simulink model "AeroModel_v2point1"  (R2021a)
settings: Solver=ode4  StartTime=0.0  StopTime=10.0  FixedStep=0.0001  RelTol=1e-3
settings Model: Creator=jadg1  LastModifiedBy=jadg1

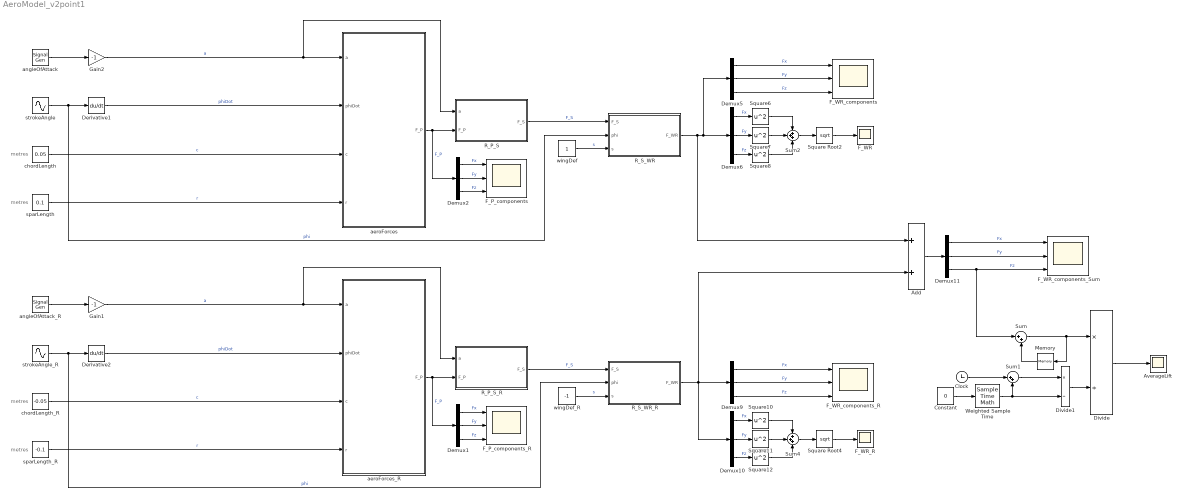
== system AeroModel_v2point1 ==
  note: metres
  note: metres
  note: metres
  note: metres
  Add : Sum
  AverageLift : Scope
  Clock : Clock
  Constant : Constant  Value=0
  Demux{1..2,5..6,9..11} (7 alike) : Demux  Outputs=3
  Derivative1 : Derivative
  Derivative2 : Derivative
  Divide : Product  Inputs=*/
  Divide1 : Product  Inputs=*/
  F_P_components : Scope  NumInputPorts=3
  F_P_components_R : Scope  NumInputPorts=3
  F_WR : Scope
  F_WR_R : Scope
  F_WR_components : Scope  NumInputPorts=3
  F_WR_components_R : Scope  NumInputPorts=3
  F_WR_components_Sum : Scope  NumInputPorts=3
  Gain1 : Gain  Gain=-1
  Gain2 : Gain  Gain=-1
  Memory : Memory
  R_P_S : MATLAB Function  TreatAsAtomicUnit=on
  R_P_S_R : MATLAB Function  TreatAsAtomicUnit=on
  R_S_WR : MATLAB Function  TreatAsAtomicUnit=on
  R_S_WR_R : MATLAB Function  TreatAsAtomicUnit=on
  Square Root2 : Sqrt  SaturateOnIntegerOverflow=on
  Square Root4 : Sqrt  SaturateOnIntegerOverflow=on
  Square{6..8,10..12} (6 alike) : Math  Operator=square  SaturateOnIntegerOverflow=on
  Sum : Sum  Inputs=|++
  Sum1 : Sum  Inputs=|++
  Sum2 : Sum  Inputs=+++
  Sum4 : Sum  Inputs=+++
  Weighted Sample Time : SampleTimeMath  TsampMathOp=Ts Only
  aeroForces : MATLAB Function  TreatAsAtomicUnit=on
  aeroForces_R : MATLAB Function  TreatAsAtomicUnit=on
  angleOfAttack : SignalGenerator  WaveForm=square  Amplitude=pi()/4  Frequency=30
  angleOfAttack_R : SignalGenerator  WaveForm=square  Amplitude=pi()/4  Frequency=30
  chordLength : Constant  Value=0.05
  chordLength_R : Constant  Value=-0.05
  sparLength : Constant  Value=0.1
  sparLength_R : Constant  Value=-0.1
  strokeAngle : Sin  Amplitude=pi()/2  Frequency=188.5  Phase=pi()/2  SampleTime=0
  strokeAngle_R : Sin  Amplitude=pi()/2  Frequency=188.5  Phase=pi()/2  SampleTime=0
  wingDef : Constant
  wingDef_R : Constant  Value=-1
  wires:
  Square11/1 -> Sum4/2
  sparLength/1 -> aeroForces/4(r)  "r"
  Demux1/3 -> F_P_components_R/3  "Fz"
  wingDef_R/1 -> R_S_WR_R/3(s)  "s"
  Derivative2/1 -> aeroForces_R/2(phiDot)  "phiDot"
  Demux10/1 -> Square10/1  "Fx"
  angleOfAttack_R/1 -> Gain1/1
  R_P_S/1(F_S) -> R_S_WR/1(F_S)  "F_S"
  Demux1/2 -> F_P_components_R/2  "Fy"
  Demux5/3 -> F_WR_components/3  "Fz"
  Demux2/3 -> F_P_components/3  "Fz"
  wingDef/1 -> R_S_WR/3(s)  "s"
  Demux10/2 -> Square11/1  "Fy"
  Gain2/1 -> R_P_S/1(a), aeroForces/1(a)  "a"
  R_S_WR_R/1(F_WR) -> Demux10/1, Demux9/1, Add/2
  Square10/1 -> Sum4/1
  Demux9/2 -> F_WR_components_R/2  "Fy"
  Sum4/1 -> Square Root4/1
  Demux10/3 -> Square12/1  "Fz"
  Square7/1 -> Sum2/2
  Demux5/1 -> F_WR_components/1  "Fx"
  Demux6/3 -> Square8/1  "Fz"
  Demux6/2 -> Square7/1  "Fy"
  Square Root2/1 -> F_WR/1
  Demux5/2 -> F_WR_components/2  "Fy"
  Demux11/2 -> F_WR_components_Sum/2  "Fy"
  Sum1/1 -> Divide1/1
  R_S_WR/1(F_WR) -> Demux6/1, Demux5/1, Add/1
  Derivative1/1 -> aeroForces/2(phiDot)  "phiDot"
  Sum/1 -> Memory/1, Divide/1
  chordLength/1 -> aeroForces/3(c)  "c"
  Square8/1 -> Sum2/3
  Divide1/1 -> Divide/2
  Demux1/1 -> F_P_components_R/1  "Fx"
  Weighted Sample Time/1 -> Sum1/2, Divide1/2
  Square Root4/1 -> F_WR_R/1
  R_P_S_R/1(F_S) -> R_S_WR_R/1(F_S)  "F_S"
  Demux9/3 -> F_WR_components_R/3  "Fz"
  sparLength_R/1 -> aeroForces_R/4(r)  "r"
  Square6/1 -> Sum2/1
  aeroForces_R/1(F_P) -> R_P_S_R/2(F_P), Demux1/1  "F_P"
  strokeAngle_R/1 -> Derivative2/1, R_S_WR_R/2(phi)  "phi"
  Sum2/1 -> Square Root2/1
  Memory/1 -> Sum/2
  Constant/1 -> Weighted Sample Time/1
  Demux2/2 -> F_P_components/2  "Fy"
  angleOfAttack/1 -> Gain2/1
  Demux11/1 -> F_WR_components_Sum/1  "Fx"
  Clock/1 -> Sum1/1
  Demux11/3 -> Sum/1, F_WR_components_Sum/3  "Fz"
  Demux9/1 -> F_WR_components_R/1  "Fx"
  Gain1/1 -> aeroForces_R/1(a), R_P_S_R/1(a)  "a"
  Demux6/1 -> Square6/1  "Fx"
  Add/1 -> Demux11/1
  Demux2/1 -> F_P_components/1  "Fx"
  strokeAngle/1 -> R_S_WR/2(phi), Derivative1/1  "phi"
  aeroForces/1(F_P) -> Demux2/1, R_P_S/2(F_P)  "F_P"
  Square12/1 -> Sum4/3
  Divide/1 -> AverageLift/1
  chordLength_R/1 -> aeroForces_R/3(c)  "c"

== matlab function AeroModel_v2point1/R_S_WR ==
  data: F_S input; phi input; s input; F_WR output
function F_WR = S_to_WR(F_S,phi,s)

arg = s*phi;

R_S_WR = [  
           cos(arg)  -sin(arg)    0 ;
           sin(arg)   cos(arg)    0 ;
              0          0        1 ;
         ];

F_WR = R_S_WR * F_S;

end

== matlab function AeroModel_v2point1/aeroForces ==
  data: a input; F_P output; phiDot input; c input; r input
function F_P = aeroForces(a,phiDot,c,r)

% Declare sizes
F_P = zeros(3,1);

% Define the density of air [kg/m^3]
p = 1.225; 

% Define the value of the F-P angle theta
theta = -a;

% Define the lift and drag coefficients using the absolute value of alpha
cL = 0.225 + 1.58*sin((2.13*abs(a))-(7.2*(pi()/180)));
cD = 1.92 - 1.55*cos((2.04*abs(a))-(9.82*(pi()/180)));

% Calculate the cartesian components of the force vector in the P frame
Fx_P = (-1/6)*cos(theta)*sign(a)*p*(phiDot^2)*cD*c*(r^3) + (1/6)*sin(theta)*p*(phiDot^2)*cL*c*(r^3);
Fy_P = 0;
Fz_P = (1/6)*sin(theta)*sign(a)*p*(phiDot^2)*cD*c*(r^3) + (1/6)*cos(theta)*p*(phiDot^2)*cL*c*(r^3);

% Construct the force vector in the P frame
F_P = [ Fx_P ;
        Fy_P ; 
        Fz_P ; ];

end

== matlab function AeroModel_v2point1/R_P_S ==
  data: a input; F_P input; F_S output
function F_S = P_to_S(a,F_P)

R_P_S = [  
           cos(a)   0   sin(a) ;
             0      1     0    ;
          -sin(a)   0   cos(a) ;
        ];

F_S = R_P_S * F_P;

end

== matlab function AeroModel_v2point1/R_P_S_R ==
  data: a input; F_P input; F_S output
function F_S = P_to_S(a,F_P)

R_P_S = [  
           cos(a)   0   sin(a) ;
             0      1     0    ;
          -sin(a)   0   cos(a) ;
        ];

F_S = R_P_S * F_P;

end

== matlab function AeroModel_v2point1/R_S_WR_R ==
  data: F_S input; phi input; s input; F_WR output
function F_WR = S_to_WR(F_S,phi,s)

arg = s*phi;

R_S_WR = [  
           cos(arg)  -sin(arg)    0 ;
           sin(arg)   cos(arg)    0 ;
              0          0        1 ;
         ];

F_WR = R_S_WR * F_S;

end

== matlab function AeroModel_v2point1/aeroForces_R ==
  data: a input; F_P output; phiDot input; c input; r input
function F_P = aeroForces(a,phiDot,c,r)

% Declare sizes
F_P = zeros(3,1);

% Define the density of air [kg/m^3]
p = 1.225; 

% Define the value of the F-P angle theta
theta = -a;

% Define the lift and drag coefficients using the absolute value of alpha
cL = 0.225 + 1.58*sin((2.13*abs(a))-(7.2*(pi()/180)));
cD = 1.92 - 1.55*cos((2.04*abs(a))-(9.82*(pi()/180)));

% Calculate the cartesian components of the force vector in the P frame
Fx_P = (-1/6)*cos(theta)*sign(a)*p*(phiDot^2)*cD*c*(r^3) + (1/6)*sin(theta)*p*(phiDot^2)*cL*c*(r^3);
Fy_P = 0;
Fz_P = (1/6)*sin(theta)*sign(a)*p*(phiDot^2)*cD*c*(r^3) + (1/6)*cos(theta)*p*(phiDot^2)*cL*c*(r^3);

% Construct the force vector in the P frame
F_P = [ Fx_P ;
        Fy_P ; 
        Fz_P ; ];

end
